simulink model "PuebaChartof"  (R2025b)
settings: Solver=VariableStepAuto  StartTime=0.0  StopTime=10.0  RelTol=1e-3

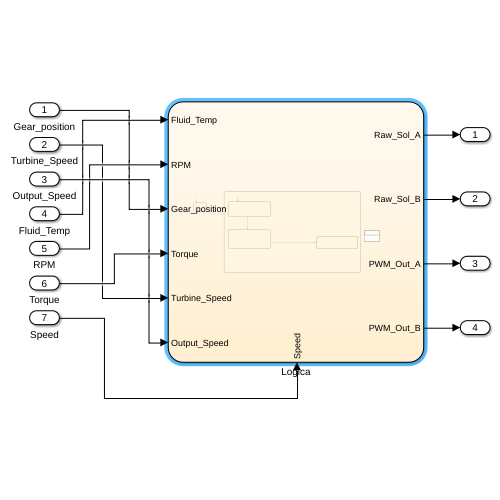
[thumbnail: Simulink's stored preview of the top-level diagram]
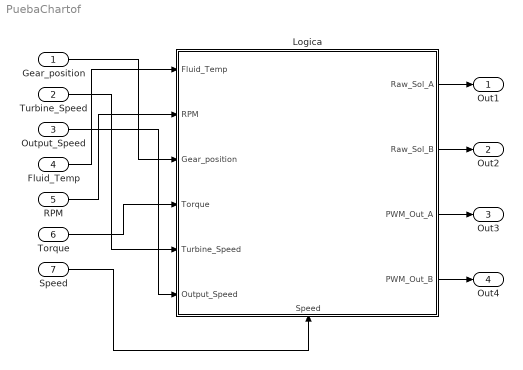
== system PuebaChartof ==
  Gear_position : Inport
  Turbine_Speed : Inport  Port=2
  Output_Speed : Inport  Port=3
  Fluid_Temp : Inport  Port=4
  RPM : Inport  Port=5
  Torque : Inport  Port=6
  Speed : Inport  Port=7
  Logica : Stateflow chart  TreatAsAtomicUnit=on
      settings: PortSchema="{\"entries\":[{\"content\":{\"sides\":[{\"content\":{\"connectorIds\":[\"In2\",\"In3\",\"In4\",\"In5\",\"In6\",\"In7\"]},\"type\":\"ConnectorPlacement.EquallySpacedRectSide\",\"uuid\":\"6f10a648-5d9c-4e67-9b7c-29cb7d46d48c\"},{\"content\":{\"connectorIds\":[\"Out1\",\"Out2\",\"Out3\",\"Out4\"],\"side\":\"RIGHT\"},\"type\":\"ConnectorPlacement.EquallySpacedRectSide\",\"uuid\":\"cb5c41a3-9c7d-4a5c-b000-08b8a55f6534\"},{\"content\":{\"side\":\"TOP\"},\"type\":\"ConnectorPlacement.EquallySpacedRectSide\",\"uuid\":\"41a50d7c-ca4f-4460-9f75-4b94977a94ef\"},{\"content\":{\"connectorIds\":[\"In1\"],\"side\":\"BOTTOM\"},\"type\":\"ConnectorPlacement.EquallySpacedRectSide\",\"uuid\":\"0d107e0b-ff30-4da8-9209-a9dfba6fd8b9\"}]},\"type\":\"ConnectorPlacement.EquallySpacedConnector\",\"uuid\":\"612f2c4e-0d90-411c-b1ad-12beb53593f0\"}],\"packageUris\":[\"http://schema.mathworks.com/mf0/Connector/R2020b\"],\"version\":\"1.0\"}"
  Out1 : Outport
  Out2 : Outport  Port=2
  Out3 : Outport  Port=3
  Out4 : Outport  Port=4
  wires:
  Gear_position/1 -> Logica/4(Gear_position)
  Fluid_Temp/1 -> Logica/2(Fluid_Temp)
  RPM/1 -> Logica/3(RPM)
  Torque/1 -> Logica/5(Torque)
  Speed/1 -> Logica/1(Speed)
  Logica/4(PWM_Out_B) -> Out4/1
  Logica/3(PWM_Out_A) -> Out3/1
  Logica/2(Raw_Sol_B) -> Out2/1
  Logica/1(Raw_Sol_A) -> Out1/1
  Output_Speed/1 -> Logica/7(Output_Speed)
  Turbine_Speed/1 -> Logica/6(Turbine_Speed)

== stateflow chart PuebaChartof/Logica ==
  state Regular
    state Marcha_1_fija
      entry:Raw_Sol_A=95; Raw_Sol_B=5;
      during:PWM_Out_A=Regulas_Salidas(Raw_Sol_A);
      PWM_Out_B=Regulas_Salidas(Raw_Sol_B);
    state Cambio_1_a_2
      entry:cnt=0; Target_S2=90;
      during: cnt=cnt+1;
      if cnt<10 Raw_Sol_A=95; Raw_Sol_B=90;
      else Raw_Sol_A = 95 - ((cnt - 10)*2);
      Raw_Sol_B=20 + ((cnt - 10)*1.5)+(Torque*0.1);
      end;
      PWM_Out_A=Regulas_Salidas(Raw_Sol_A);
      PWM_Out_B=Regulas_Salidas(Raw_Sol_B);
    state Marcha_2_Fija
      entry: Raw_Sol_A=0; Raw_Sol_B=95;
      during:PWM_Out_A=Regulas_Salidas(Raw_Sol_A);
      PWM_Out_B=Regulas_Salidas(Raw_Sol_B);
    (default) -> Marcha_1_fija
    Marcha_1_fija -> Cambio_1_a_2 : [Speed>20 &&Torque < 60 ]
    Cambio_1_a_2 -> Marcha_2_Fija : [Turbine_Speed<(Output_Speed*Ratio_2)]
  state Reposo
  (default) -> Reposo
  Reposo -> Regular : [Gear_position==1]
  data: Raw_input function_input; pwm_limpio function_output; Raw_Sol_A output; Raw_Sol_B output; PWM_Out_A output; Speed input; Fluid_Temp input; RPM input; Gear_position input; Torque input; PWM_Out_B output; cnt local; Turbine_Speed input; Output_Speed input; Ratio_2 constant double =1.5; Target_S2 local
  function pwm_limpio = Regulas_Salidas(Raw_input):
    | function pwm_limpio = Regulas_Salidas(Raw_input)
    |     if Raw_input > 95
    |         pwm_limpio = 95;
    |     elseif Raw_input < 5
    |         pwm_limpio = 5;
    |     else 
    |         pwm_limpio = Raw_input;
    |     end
